simulink model "problem2"  (R2020b)
settings: Solver=VariableStepAuto  StartTime=0.0  StopTime=100.0  RelTol=1e-3
values from neighbouring files (symbols this model uses):
  b = 350    [variables.m]
  k1 = 80000    [variables.m]
  k2 = 500000    [variables.m]
  M1 = 2500    [variables.m]
  M2 = 320    [variables.m]
settings Model: Creator=shweta  LastModifiedBy=shweta

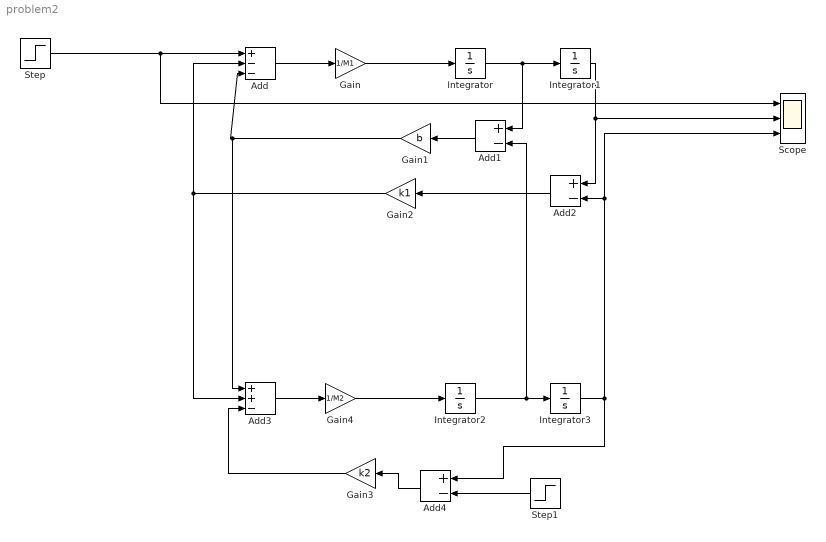
== system problem2 ==
  Add : Sum  Inputs=+--
  Add1 : Sum  Inputs=+-
  Add2 : Sum  Inputs=+-
  Add3 : Sum  Inputs=++-
  Add4 : Sum  Inputs=+-
  Gain : Gain  Gain=1/M1
  Gain1 : Gain  Gain=b
  Gain2 : Gain  Gain=k1
  Gain3 : Gain  Gain=k2
  Gain4 : Gain  Gain=1/M2
  Integrator{,1..3} (4 alike) : Integrator
  Scope : Scope  NumInputPorts=3
  Step : Step  After=5  SampleTime=0
  Step1 : Step  After=15  SampleTime=0
  wires:
  Add/1 -> Gain/1
  Gain/1 -> Integrator/1
  Integrator/1 -> Add1/1, Integrator1/1
  Add3/1 -> Gain4/1
  Integrator2/1 -> Add1/2, Integrator3/1
  Gain4/1 -> Integrator2/1
  Add1/1 -> Gain1/1
  Integrator1/1 -> Add2/1, Scope/2
  Add2/1 -> Gain2/1
  Gain2/1 -> Add3/2, Add/2
  Gain1/1 -> Add3/1, Add/3
  Add4/1 -> Gain3/1
  Gain3/1 -> Add3/3
  Integrator3/1 -> Scope/3, Add2/2, Add4/1
  Step/1 -> Scope/1, Add/1
  Step1/1 -> Add4/2
